simulink model "model_simulink"  (R2017b)
settings: Solver=ode8  StartTime=0.0  StopTime=100  FixedStep=0.01  MaxStep=8.0  RelTol=1e-3
undefined symbols (not defined in the file): Serial_Port, Standard_Devices
libraries: simulink x3, sldrtlib x2
settings Model: Creator=Vjekoslav  LastModifiedBy=Vjekoslav
settings CodeAppCC: StateflowObjectComments=on

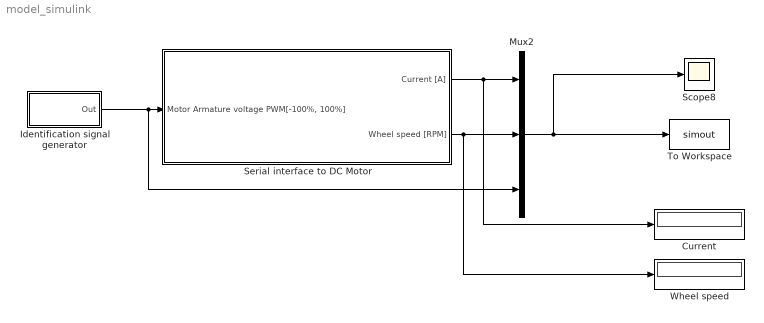
== system model_simulink ==
  Current : Display
  Identification signal generator : Subsystem
  Mux2 : Mux  Inputs=3
  Scope8 : Scope
  "Serial interface to DC Motor " : Subsystem
  To Workspace : ToWorkspace  VariableName=simout  SaveFormat=Timeseries  SampleTime=-1
  Wheel speed : Display
  wires:
  Mux2/1 -> Scope8/1, To Workspace/1
  "Serial interface to DC Motor "/1(Current [A]) -> Mux2/1, Current/1
  "Serial interface to DC Motor "/2(Wheel speed [RPM]) -> Mux2/2, Wheel speed/1
  Identification signal generator/1(Out) -> Mux2/3, "Serial interface to DC Motor "/1("Motor Armature voltage PWM[-100%, 100%] ")

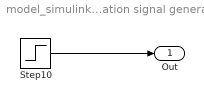
== system model_simulink/Identification signal generator ==
  Step10 : Step  Time=5  Before=40  After=60  SampleTime=0
  Out : Outport
  wires:
  Step10/1 -> Out/1

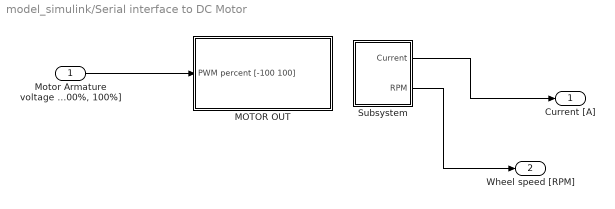
== system model_simulink/Serial interface to DC Motor  ==
  "Motor Armature voltage PWM[-100%, 100%] " : Inport
  MOTOR OUT : Subsystem
  Subsystem : Subsystem
  Current [A] : Outport
  Wheel speed [RPM] : Outport  Port=2
  wires:
  "Motor Armature voltage PWM[-100%, 100%] "/1 -> MOTOR OUT/1(PWM percent [-100 100])
  Subsystem/1(Current) -> Current [A]/1
  Subsystem/2("RPM ") -> Wheel speed [RPM]/1

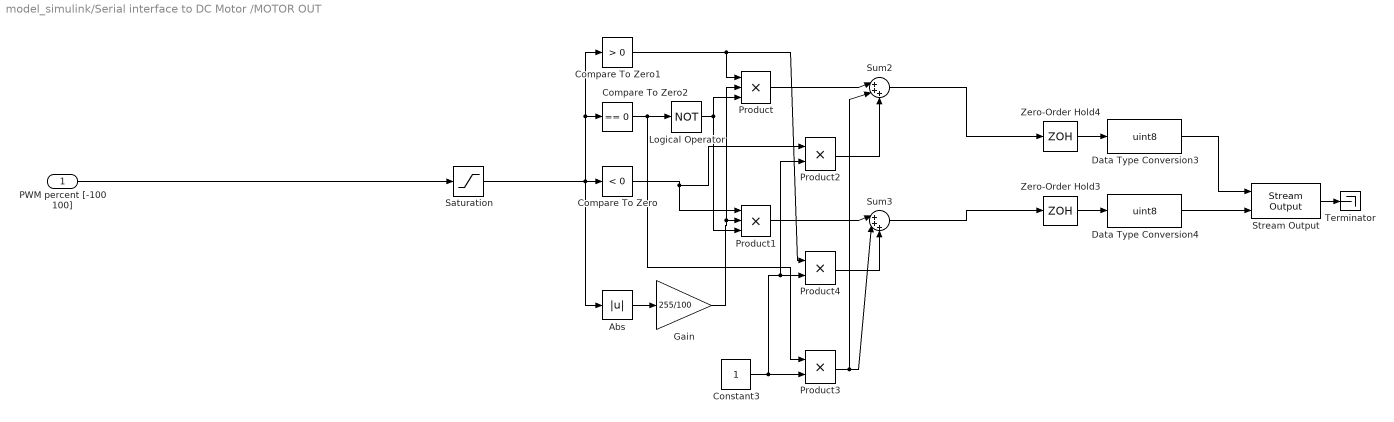
== system model_simulink/Serial interface to DC Motor /MOTOR OUT ==
  PWM percent [-100 100] : Inport
  Abs : Abs
  Compare To Zero : simulink/Logic and Bit Operations/Compare To Zero  relop=<  OutDataTypeStr=boolean
  Compare To Zero1 : simulink/Logic and Bit Operations/Compare To Zero  relop=>  OutDataTypeStr=boolean
  Compare To Zero2 : simulink/Logic and Bit Operations/Compare To Zero  relop===  OutDataTypeStr=boolean
  Constant3 : Constant
  Data Type Conversion3 : DataTypeConversion  OutMin=[0]  OutMax=[255]  OutDataTypeStr=uint8  RndMeth=Nearest
  Data Type Conversion4 : DataTypeConversion  OutMin=[0]  OutMax=[255]  OutDataTypeStr=uint8  RndMeth=Nearest
  Gain : Gain  Gain=255/100
  Logical Operator : Logic  Operator=NOT  AllPortsSameDT=off  OutDataTypeStr=boolean
  Product : Product  Inputs=3
  Product1 : Product  Inputs=3
  Product2 : Product
  Product3 : Product
  Product4 : Product
  Saturation : Saturate  UpperLimit=100  LowerLimit=-100
  Stream Output : sldrtlib/Stream Output  SampleTime=-1  MaxMissedTicks=inf  ShowMissedTicks=off  YieldWhenWaiting=off  DrvName=Standard_Devices/Serial_Port  DrvAddress=4  DrvOptions=[1000000 8 0 0 0 0 0 0]  PortSizes=[1 1]  FormatString='%c%c\n'  ShowReady=off  ShowError=on  InitialValue=[]  FinalValue=[]
      settings: AttributesFormatString=Standard Devices\nSerial Port [4h]  SourceProductName=Simulink Desktop Real-Time  SourceProductBaseCode=WT
  Sum2 : Sum  Inputs=|+++
  Sum3 : Sum  Inputs=|+++
  Terminator : Terminator
  Zero-Order Hold3 : ZeroOrderHold  SampleTime=-1
  Zero-Order Hold4 : ZeroOrderHold  SampleTime=-1
  wires:
  Product4/1 -> Sum3/3
  Product2/1 -> Sum2/3
  Logical Operator/1 -> Product/3, Product1/3
  Compare To Zero2/1 -> Product3/1, Logical Operator/1
  Product1/1 -> Sum3/1
  Sum3/1 -> Zero-Order Hold3/1
  Constant3/1 -> Product2/2, Product4/2, Product3/2
  Saturation/1 -> Abs/1, Compare To Zero1/1, Compare To Zero2/1, Compare To Zero/1
  Product3/1 -> Sum3/2, Sum2/2
  Compare To Zero1/1 -> Product4/1, Product/1
  Data Type Conversion3/1 -> Stream Output/1
  Zero-Order Hold3/1 -> Data Type Conversion4/1
  Gain/1 -> Product1/2, Product/2
  Abs/1 -> Gain/1
  Sum2/1 -> Zero-Order Hold4/1
  Zero-Order Hold4/1 -> Data Type Conversion3/1
  Compare To Zero/1 -> Product2/1, Product1/1
  Product/1 -> Sum2/1
  Data Type Conversion4/1 -> Stream Output/2
  Stream Output/1 -> Terminator/1
  PWM percent [-100 100]/1 -> Saturation/1

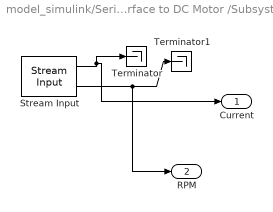
== system model_simulink/Serial interface to DC Motor /Subsystem ==
  Stream Input : sldrtlib/Stream Input  SampleTime=-1  MaxMissedTicks=inf  ShowMissedTicks=off  YieldWhenWaiting=off  DrvName=Standard_Devices/Serial_Port  DrvAddress=4  DrvOptions=[1000000 8 0 0 0 0 0 0]  DataTypes={ 'double' 'double'}  FormatString='\r%f\r%f'  Terminator='\n'  ShowReady=off  ShowError=off
      settings: AttributesFormatString=Serial Port [4]  SourceProductName=Simulink Desktop Real-Time  SourceProductBaseCode=WT
  Terminator : Terminator
  Terminator1 : Terminator
  Current : Outport
  "RPM " : Outport  Port=2
  wires:
  Stream Input/1 -> Current/1, Terminator/1
  Stream Input/2 -> "RPM "/1, Terminator1/1
